simulink model "WindTurbineESCKOpt"  (R2021a)
settings: Solver=VariableStepDiscrete  StartTime=0.0  StopTime=inf  MaxStep=Ts  RelTol=1e-3
undefined symbols (not defined in the file): K_i, T, Ts
libraries: DRC_SimulinkLibrary x2
settings Model: PacingRate=79  Creator=Sebastiaan  LastModifiedBy=Sebastiaan

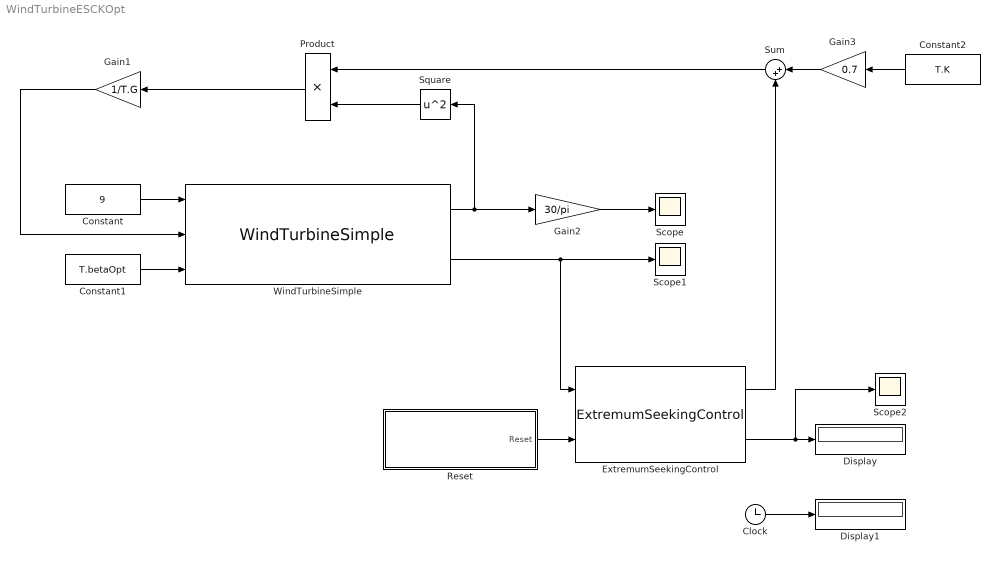
== system WindTurbineESCKOpt ==
  Clock : Clock
  Constant : Constant  Value=9
  Constant1 : Constant  Value=T.betaOpt
  Constant2 : Constant  Value=T.K
  Display : Display
  Display1 : Display
  ExtremumSeekingControl : DRC_SimulinkLibrary/ExtremumSeekingControl  D_A=D_A  D_w=D_w  M_phi=M_phi  Ki=K_i  LPF_wc=wc_LPF  HPF_wc=wc_HPF  Ts=Ts
  Gain1 : Gain  Gain=1/T.G
  Gain2 : Gain  Gain=30/pi
  Gain3 : Gain  Gain=0.7
  Product : Product
  Reset : Subsystem
  Scope : Scope
  Scope1 : Scope
  Scope2 : Scope
  Square : Math  Operator=square  SaturateOnIntegerOverflow=on
  Sum : Sum  Inputs=|++
  WindTurbineSimple : DRC_SimulinkLibrary/WindTurbineSimple  R=T.R  rho=T.rho  TMax=inf  JWr=T.Jlss  G=T.G  Wr0=Wr0  CpArray=T.Cp  TSRVec=T.CTSR  betaVec=T.CPitch
  wires:
  Constant/1 -> WindTurbineSimple/1
  Constant1/1 -> WindTurbineSimple/3
  Gain2/1 -> Scope/1
  WindTurbineSimple/1 -> Gain2/1, Square/1
  Gain1/1 -> WindTurbineSimple/2
  Product/1 -> Gain1/1
  WindTurbineSimple/2 -> ExtremumSeekingControl/1, Scope1/1
  Square/1 -> Product/2
  Constant2/1 -> Gain3/1
  Gain3/1 -> Sum/1
  Sum/1 -> Product/1
  ExtremumSeekingControl/2 -> Scope2/1, Display/1
  ExtremumSeekingControl/1 -> Sum/2
  Reset/1(Reset) -> ExtremumSeekingControl/2
  Clock/1 -> Display1/1

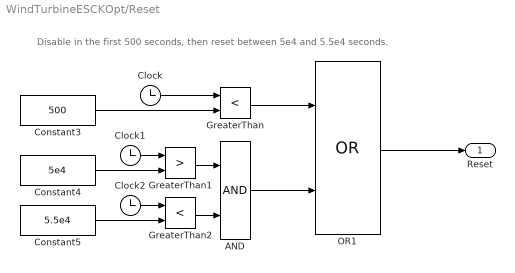
== system WindTurbineESCKOpt/Reset ==
  note: Disable in the first 500 seconds, then reset between 5e4 and 5.5e4 seconds.
  AND : Logic  AllPortsSameDT=off  OutDataTypeStr=boolean
  Clock : Clock
  Clock1 : Clock
  Clock2 : Clock
  Constant3 : Constant  Value=500
  Constant4 : Constant  Value=5e4
  Constant5 : Constant  Value=5.5e4
  GreaterThan : RelationalOperator  Operator=<  OutDataTypeStr=boolean  RndMeth=Simplest
  GreaterThan1 : RelationalOperator  Operator=>  OutDataTypeStr=boolean  RndMeth=Simplest
  GreaterThan2 : RelationalOperator  Operator=<  OutDataTypeStr=boolean  RndMeth=Simplest
  OR1 : Logic  Operator=OR  AllPortsSameDT=off  OutDataTypeStr=boolean
  Reset : Outport
  wires:
  Clock1/1 -> GreaterThan1/1
  GreaterThan1/1 -> AND/1
  Clock2/1 -> GreaterThan2/1
  AND/1 -> OR1/2
  GreaterThan/1 -> OR1/1
  Constant3/1 -> GreaterThan/2
  Constant4/1 -> GreaterThan1/2
  Constant5/1 -> GreaterThan2/2
  GreaterThan2/1 -> AND/2
  Clock/1 -> GreaterThan/1
  OR1/1 -> Reset/1
